simulink model "double_sim"  (R2022b)
settings: Solver=VariableStepAuto  StartTime=0.0  StopTime=7  RelTol=1e-3
values from neighbouring files (symbols this model uses):
  dt = 0.005    [double_main.m]    (also in double_main_px4.m; double_main_so3.m; se3controller.m = 0.001)
  J = diag([0.082,0.0845,0.1377])/2.5/2.5/4.34*m    [double_main.m]    (also in double_main_px4.m = diag([0.0031 0.0032 0.0045]); double_main_so3.m = diag([0.0031 0.0032 0.0045]); my_exp1.m = diag([Ixx,Iyy,Izz]))
  K = lqr(sys,Q,R)    [double_main.m]    (also in double_main_px4.m; double_main_so3.m)
  kv = m*K(1,4)    [double_main.m]    (also in double_main_px4.m = m*K1(1,4); double_main_so3.m = m*K1(1,4); se3controller.m = 2)
  kx = m*K(1,1)    [double_main.m]    (also in double_main_px4.m = m*K1(1,1); double_main_so3.m = m*K1(1,1); se3controller.m = 3)
  m = 0.8    [double_main.m]    (also in double_main_px4.m = 0.8771; double_main_so3.m = 0.8771; my_exp1.m; run_exp1.m = 0.5)
libraries: shared6dof x1, aerolibutil x1
settings Model: Creator=zzy  LastModifiedBy=zzy
settings DataIOCC: ReturnWorkspaceOutputs=off

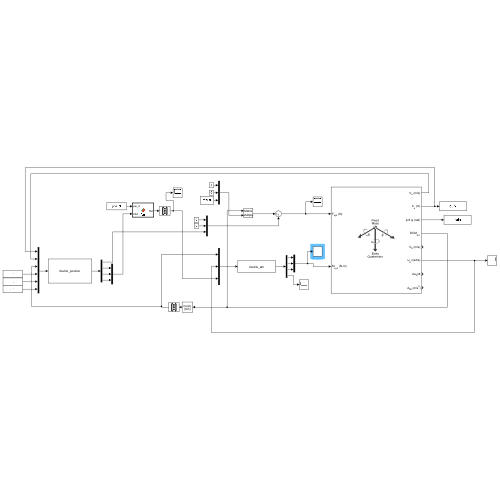
[thumbnail: Simulink's stored preview of the top-level diagram]
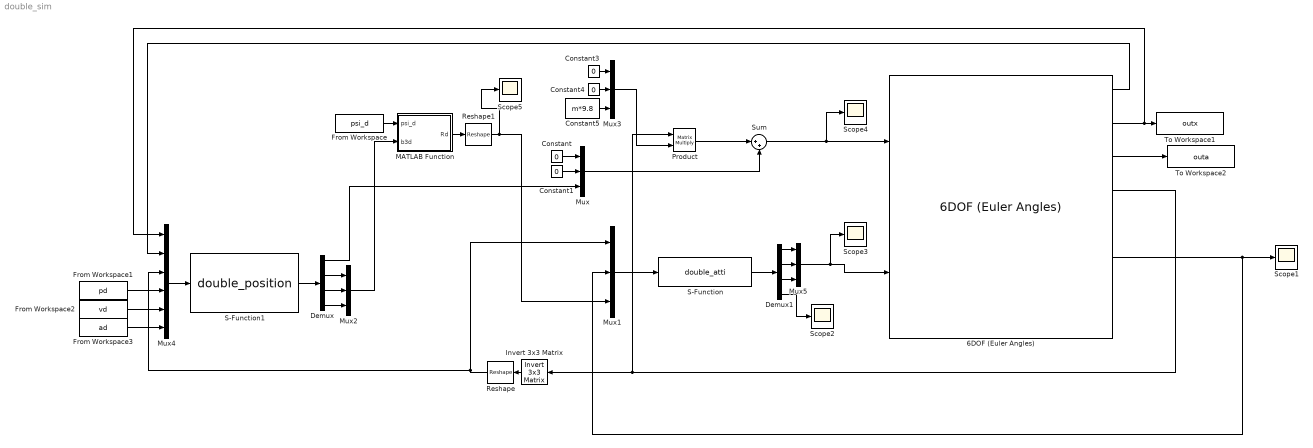
== system double_sim ==
  6DOF (Euler Angles) : shared6dof/6DOF (Euler Angles)  units=Metric (MKS)  mtype=Fixed  rep=Quaternion  xme_0=[0 0 0]  Vm_0=[0 0 0]  eul_0=[0 0 0]  pm_0=[0 0 0]  mass_0=1  mass_e=0.5  mass_f=2.0  inertia=J  inertia_e=eye(3)  inertia_f=2*eye(3)  k_quat=1.0  vre_flag=on  abi_flag=off  aMode=0  xme_statename=''  Vm_statename=''  eul_statename=''  quat_statename=''  pm_statename=''  mass_statename=''
  Constant{,1,3..4} (4 alike) : Constant  Value=0
  Constant5 : Constant  Value=m*9.8
  Demux : Demux
  Demux1 : Demux
  From Workspace : FromWorkspace  VariableName=psi_d
  From Workspace1 : FromWorkspace  VariableName=pd
  From Workspace2 : FromWorkspace  VariableName=vd
  From Workspace3 : FromWorkspace  VariableName=ad
  Invert 3x3 Matrix : aerolibutil/Invert  3x3 Matrix
  MATLAB Function : MATLAB Function  TreatAsAtomicUnit=on
  Mux{,1..3,5} (5 alike) : Mux  Inputs=3
  Mux4 : Mux  Inputs=6
  Product : Product  Multiplication=Matrix(*)
  Reshape : Reshape  OutputDimensionality=Column vector (2-D)
  Reshape1 : Reshape  OutputDimensionality=Column vector (2-D)
  S-Function : S-Function  FunctionName=double_atti  Parameters=dt,J,K  SFunctionDeploymentMode=off  EnableBusSupport=off
  S-Function1 : S-Function  FunctionName=double_position  Parameters=dt,m,kx,kv  SFunctionDeploymentMode=off  EnableBusSupport=off
  Scope{1..5} (5 alike) : Scope
  Sum : Sum  Inputs=|++
  To Workspace1 : ToWorkspace  VariableName=outx  SampleTime=-1
      settings: Save2DSignal=2-D array (concatenate along first dimension)
  To Workspace2 : ToWorkspace  VariableName=outa  SampleTime=-1
      settings: Save2DSignal=2-D array (concatenate along first dimension)
  wires:
  Constant1/1 -> Mux/2
  Constant/1 -> Mux/1
  6DOF (Euler Angles)/6 -> Mux1/2, Scope1/1
  Invert 3x3 Matrix/1 -> Reshape/1
  Mux1/1 -> S-Function/1
  Reshape/1 -> Mux1/1, Mux4/3
  6DOF (Euler Angles)/3 -> To Workspace2/1
  From Workspace/1 -> MATLAB Function/1(psi_d)
  MATLAB Function/1(Rd) -> Reshape1/1
  Demux/2 -> Mux2/1
  Demux/4 -> Mux2/3
  Demux/3 -> Mux2/2
  S-Function1/1 -> Demux/1
  Mux2/1 -> MATLAB Function/2(b3d)
  6DOF (Euler Angles)/4 -> Product/1, Invert 3x3 Matrix/1
  Constant3/1 -> Mux3/1
  Mux3/1 -> Product/2
  Constant4/1 -> Mux3/2
  Constant5/1 -> Mux3/3
  Product/1 -> Sum/1
  Demux/1 -> Mux/3
  Mux/1 -> Sum/2
  Sum/1 -> Scope4/1, 6DOF (Euler Angles)/1
  6DOF (Euler Angles)/2 -> To Workspace1/1, Mux4/1
  6DOF (Euler Angles)/1 -> Mux4/2
  From Workspace1/1 -> Mux4/4
  From Workspace2/1 -> Mux4/5
  From Workspace3/1 -> Mux4/6
  Mux4/1 -> S-Function1/1
  Reshape1/1 -> Scope5/1, Mux1/3
  S-Function/1 -> Demux1/1
  Demux1/1 -> Mux5/1
  Demux1/2 -> Mux5/2
  Demux1/3 -> Mux5/3
  Mux5/1 -> Scope3/1, 6DOF (Euler Angles)/2
  Demux1/4 -> Scope2/1

== matlab function double_sim/MATLAB Function ==
  data: psi_d input; Rd output; b3d input
function Rd = fcn(psi_d,b3d)
b1d=[cos(psi_d);sin(psi_d);0];
b2d=cross(b3d,b1d)/norm(cross(b3d,b1d));
Rd=[cross(b2d,b3d),b2d,b3d];
end
